simulink model "part_1"  (R2017b)
settings: Solver=VariableStepAuto  StartTime=0.0  StopTime=10.0  MaxStep=0.001  RelTol=1e-3
settings Model: Creator=drone  LastModifiedBy=drone

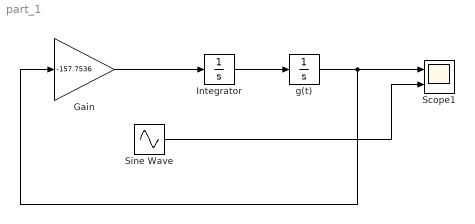
== system part_1 ==
  Gain : Gain  Gain=-157.7536
  Integrator : Integrator  InitialCondition=0.444974
  Scope1 : Scope  NumInputPorts=2
  Sine Wave : Sin  Amplitude=0.035428  Frequency=12.56  SampleTime=0
  g(t) : Integrator
  wires:
  Gain/1 -> Integrator/1
  Integrator/1 -> g(t)/1
  g(t)/1 -> Scope1/1, Gain/1
  Sine Wave/1 -> Scope1/2
